simulink model "code_gen_man_bin_test"  (Simulink 7.5)
settings: Solver=FixedStepDiscrete  StartTime=0.0  StopTime=15  RelTol=1e-3
libraries: simulink x3
settings Model: Creator=Bryant  LastModifiedBy=Bryant

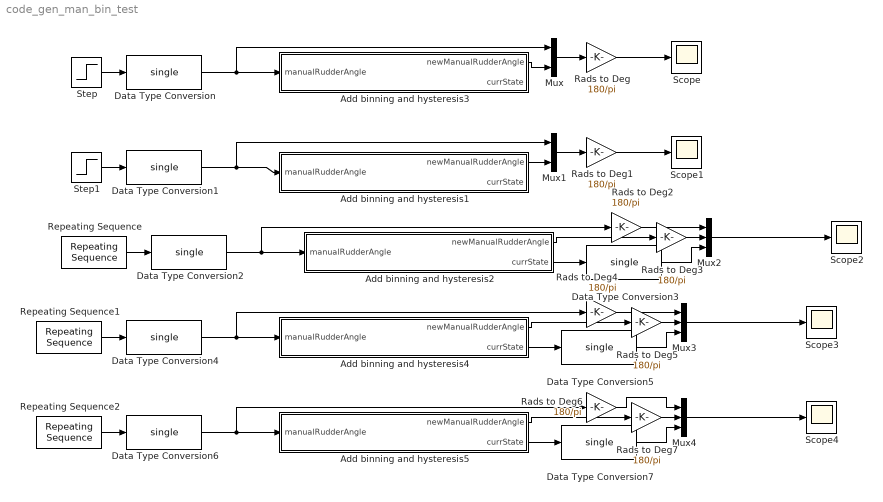
== system code_gen_man_bin_test ==
  Add binning and hysteresis1 : Stateflow chart  TreatAsAtomicUnit=on
  Add binning and hysteresis2 : Stateflow chart  TreatAsAtomicUnit=on
  Add binning and hysteresis3 : Stateflow chart  TreatAsAtomicUnit=on
  Add binning and hysteresis4 : Stateflow chart  TreatAsAtomicUnit=on
  Add binning and hysteresis5 : Stateflow chart  TreatAsAtomicUnit=on
  Data Type Conversion{,1..7} (8 alike) : DataTypeConversion  OutDataTypeMode=single  OutDataType=fixdt(1, 16)  OutScaling=2^0  OutDataTypeStr=single
  Mux : Mux  Inputs=2
  Mux1 : Mux  Inputs=2
  Mux2 : Mux  Inputs=3
  Mux3 : Mux  Inputs=3
  Mux4 : Mux  Inputs=3
  Rads to Deg{,1..7} (8 alike) : Gain  Gain=180/pi  ParameterDataType=fixdt(1, 16)  ParameterScaling=2^0  OutDataType=fixdt(1, 16)  OutScaling=2^0
  Repeating Sequence : simulink/Sources/Repeating Sequence  SystemSampleTime=-1  rep_seq_t=[0 1 1 2 2]  rep_seq_y=[0 0 35 35 0]*pi/180
  Repeating Sequence1 : simulink/Sources/Repeating Sequence  SystemSampleTime=-1  rep_seq_t=[0 1 1 2 2]  rep_seq_y=[0 0 -35 -35 0]*pi/180
  Repeating Sequence2 : simulink/Sources/Repeating Sequence  SystemSampleTime=-1  rep_seq_t=[0 1 1 2 2 3 3 4 4 5 5 6 6]  rep_seq_y=[0 0 -35 -35 0 0 35 35 0 0 -35 -35 0]*pi/180
  Scope{,1..4} (5 alike) : Scope
      Scope2 settings: SaveName=ScopeData2
      Scope3 settings: SaveName=ScopeData3
      Scope4 settings: SaveName=ScopeData4
  Step : Step  After=35*pi/180  SampleTime=.01
  Step1 : Step  After=-35*pi/180  SampleTime=.01
  wires:
  Step/1 -> Data Type Conversion/1
  Add binning and hysteresis3/1(newManualRudderAngle) -> Mux/2
  Mux/1 -> Rads to Deg/1
  Data Type Conversion/1 -> Mux/1, Add binning and hysteresis3/1(manualRudderAngle)
  Rads to Deg/1 -> Scope/1
  Step1/1 -> Data Type Conversion1/1
  Add binning and hysteresis1/1(newManualRudderAngle) -> Mux1/2
  Mux1/1 -> Rads to Deg1/1
  Data Type Conversion1/1 -> Mux1/1, Add binning and hysteresis1/1(manualRudderAngle)
  Rads to Deg1/1 -> Scope1/1
  Add binning and hysteresis2/1(newManualRudderAngle) -> Rads to Deg3/1
  Mux2/1 -> Scope2/1
  Data Type Conversion2/1 -> Add binning and hysteresis2/1(manualRudderAngle), Rads to Deg2/1
  Repeating Sequence/1 -> Data Type Conversion2/1
  Add binning and hysteresis2/2(currState) -> Data Type Conversion3/1
  Data Type Conversion3/1 -> Mux2/3
  Rads to Deg2/1 -> Mux2/1
  Rads to Deg3/1 -> Mux2/2
  Add binning and hysteresis4/1(newManualRudderAngle) -> Rads to Deg5/1
  Mux3/1 -> Scope3/1
  Data Type Conversion4/1 -> Add binning and hysteresis4/1(manualRudderAngle), Rads to Deg4/1
  Repeating Sequence1/1 -> Data Type Conversion4/1
  Add binning and hysteresis4/2(currState) -> Data Type Conversion5/1
  Data Type Conversion5/1 -> Mux3/3
  Rads to Deg4/1 -> Mux3/1
  Rads to Deg5/1 -> Mux3/2
  Add binning and hysteresis5/1(newManualRudderAngle) -> Rads to Deg7/1
  Mux4/1 -> Scope4/1
  Data Type Conversion6/1 -> Add binning and hysteresis5/1(manualRudderAngle), Rads to Deg6/1
  Repeating Sequence2/1 -> Data Type Conversion6/1
  Add binning and hysteresis5/2(currState) -> Data Type Conversion7/1
  Data Type Conversion7/1 -> Mux4/3
  Rads to Deg7/1 -> Mux4/2
  Rads to Deg6/1 -> Mux4/1

== matlab function Add binning and hysteresis1 ==
  data: manualRudderAngle input double; newManualRudderAngle output double; currState output double
function [newManualRudderAngle,currState] = fcn(manualRudderAngle)
%#eml
    % This function converts the continuous input of the rudder angle
    % command into a up/down/no change control. This allows for the commanded
    % rudder value to remain constant, which is useful for doing rudder
    % tests.
    
    % Once the input is above 25 or below -25 degrees (in radians) then a
    % counter starts for 25 timesteps (so .25s total) to see if the rudder
    % angle should change. Then it waits until the commanded angle resets
    % to around 0 (between +- 10 degrees) and then another transition can
    % occur.
    
    % This function relies on a 4-state FSM. It follows the general pattern
    % of 0-1-3 or 0-2-3 on success. 0 is the initial state, 1 and 2 are the
    % same, just moving in different directions, and 3 is the cleanup.

    % Keep a counter going of how long they have requested a bin transition
    persistent transitionCounter state nullTransitionCounter;
    if isempty(transitionCounter)
        transitionCounter = uint8(0);
        nullTransitionCounter = uint8(0);
        state = uint8(0);
    end

    % Store the mapped rudder angles for each bin
    binAngles = single([-45 -33 -22 -11 0 11 22 33 45]*pi/180);

    % Keep track of which bin we're in so that hysteresis can be done. This is
    % NOT a stateless algorithm. We initialize into the 0th bin (which is 1 in
    % this case because of Matlab's 1 indexing).
    persistent bin;
    if isempty(bin)
        bin = uint8(5);
    end

    switch state
        case 0
            if manualRudderAngle > 25*pi/180;
                transitionCounter = uint8(0);
                state = uint8(1);
            elseif manualRudderAngle < -25*pi/180;
                transitionCounter = uint8(0);
                state = uint8(2);
            end
        case 1
            % If the user is still indicating a transition, keep counting.
            % Otherwise record null transition commands.
            if manualRudderAngle > 25*pi/180;
                transitionCounter = transitionCounter + uint8(1);
            else
                nullTransitionCounter = nullTransitionCounter + uint8(1);
            end
            
            % Either transition if possible and requested or fail out after
            % having encountered too many timesteps without a request.
            if transitionCounter > 25
                if bin + uint8(1) <= length(binAngles)
                    bin = bin + uint8(1);
                end
                state = uint8(3);
            elseif nullTransitionCounter > 8
                state = uint8(3);
            end
        case 2
            if manualRudderAngle < -25*pi/180;
                transitionCounter = transitionCounter + uint8(1);
            else
                nullTransitionCounter = nullTransitionCounter + uint8(1);
            end
            if transitionCounter > 25
                if bin - uint8(1) > 0
                    bin = bin - uint8(1);
                end
                state = uint8(3);
            elseif nullTransitionCounter > 8
                state = uint8(3);
            end
        case 3
            if manualRudderAngle < 10*pi/180 && manualRudderAngle > -10*pi/180
                state = uint8(0);
                nullTransitionCounter = uint8(0);
            end
    end
    
    newManualRudderAngle = binAngles(bin);
    currState = state;
end

== matlab function Add binning and hysteresis2 ==
  data: manualRudderAngle input double; newManualRudderAngle output double; currState output double
function [newManualRudderAngle,currState] = fcn(manualRudderAngle)
%#eml
    % This function converts the continuous input of the rudder angle
    % command into a up/down/no change control. This allows for the commanded
    % rudder value to remain constant, which is useful for doing rudder
    % tests.
    
    % Once the input is above 25 or below -25 degrees (in radians) then a
    % counter starts for 25 timesteps (so .25s total) to see if the rudder
    % angle should change. Then it waits until the commanded angle resets
    % to around 0 (between +- 10 degrees) and then another transition can
    % occur.
    
    % This function relies on a 4-state FSM. It follows the general pattern
    % of 0-1-3 or 0-2-3 on success. 0 is the initial state, 1 and 2 are the
    % same, just moving in different directions, and 3 is the cleanup.

    % Keep a counter going of how long they have requested a bin transition
    persistent transitionCounter state nullTransitionCounter;
    if isempty(transitionCounter)
        transitionCounter = uint8(0);
        nullTransitionCounter = uint8(0);
        state = uint8(0);
    end

    % Store the mapped rudder angles for each bin
    binAngles = single([-45 -33 -22 -11 0 11 22 33 45]*pi/180);

    % Keep track of which bin we're in so that hysteresis can be done. This is
    % NOT a stateless algorithm. We initialize into the 0th bin (which is 1 in
    % this case because of Matlab's 1 indexing).
    persistent bin;
    if isempty(bin)
        bin = uint8(5);
    end

    switch state
        case 0
            if manualRudderAngle > 25*pi/180;
                transitionCounter = uint8(0);
                state = uint8(1);
            elseif manualRudderAngle < -25*pi/180;
                transitionCounter = uint8(0);
                state = uint8(2);
            end
        case 1
            % If the user is still indicating a transition, keep counting.
            % Otherwise record null transition commands.
            if manualRudderAngle > 25*pi/180;
                transitionCounter = transitionCounter + uint8(1);
            else
                nullTransitionCounter = nullTransitionCounter + uint8(1);
            end
            
            % Either transition if possible and requested or fail out after
            % having encountered too many timesteps without a request.
            if transitionCounter > 25
                if bin + uint8(1) <= length(binAngles)
                    bin = bin + uint8(1);
                end
                state = uint8(3);
            elseif nullTransitionCounter > 8
                state = uint8(3);
            end
        case 2
            if manualRudderAngle < -25*pi/180;
                transitionCounter = transitionCounter + uint8(1);
            else
                nullTransitionCounter = nullTransitionCounter + uint8(1);
            end
            if transitionCounter > 25
                if bin - uint8(1) > 0
                    bin = bin - uint8(1);
                end
                state = uint8(3);
            elseif nullTransitionCounter > 8
                state = uint8(3);
            end
        case 3
            if manualRudderAngle < 10*pi/180 && manualRudderAngle > -10*pi/180
                state = uint8(0);
                nullTransitionCounter = uint8(0);
            end
    end
    
    newManualRudderAngle = binAngles(bin);
    currState = state;
end

== matlab function Add binning and hysteresis3 ==
  data: manualRudderAngle input double; newManualRudderAngle output double; currState output double
function [newManualRudderAngle,currState] = fcn(manualRudderAngle)
%#eml
    % This function converts the continuous input of the rudder angle
    % command into a up/down/no change control. This allows for the commanded
    % rudder value to remain constant, which is useful for doing rudder
    % tests.
    
    % Once the input is above 25 or below -25 degrees (in radians) then a
    % counter starts for 25 timesteps (so .25s total) to see if the rudder
    % angle should change. Then it waits until the commanded angle resets
    % to around 0 (between +- 10 degrees) and then another transition can
    % occur.
    
    % This function relies on a 4-state FSM. It follows the general pattern
    % of 0-1-3 or 0-2-3 on success. 0 is the initial state, 1 and 2 are the
    % same, just moving in different directions, and 3 is the cleanup.

    % Keep a counter going of how long they have requested a bin transition
    persistent transitionCounter state nullTransitionCounter;
    if isempty(transitionCounter)
        transitionCounter = uint8(0);
        nullTransitionCounter = uint8(0);
        state = uint8(0);
    end

    % Store the mapped rudder angles for each bin
    binAngles = single([-45 -33 -22 -11 0 11 22 33 45]*pi/180);

    % Keep track of which bin we're in so that hysteresis can be done. This is
    % NOT a stateless algorithm. We initialize into the 0th bin (which is 1 in
    % this case because of Matlab's 1 indexing).
    persistent bin;
    if isempty(bin)
        bin = uint8(5);
    end

    switch state
        case 0
            if manualRudderAngle > 25*pi/180;
                transitionCounter = uint8(0);
                state = uint8(1);
            elseif manualRudderAngle < -25*pi/180;
                transitionCounter = uint8(0);
                state = uint8(2);
            end
        case 1
            % If the user is still indicating a transition, keep counting.
            % Otherwise record null transition commands.
            if manualRudderAngle > 25*pi/180;
                transitionCounter = transitionCounter + uint8(1);
            else
                nullTransitionCounter = nullTransitionCounter + uint8(1);
            end
            
            % Either transition if possible and requested or fail out after
            % having encountered too many timesteps without a request.
            if transitionCounter > 25
                if bin + uint8(1) <= length(binAngles)
                    bin = bin + uint8(1);
                end
                state = uint8(3);
            elseif nullTransitionCounter > 8
                state = uint8(3);
            end
        case 2
            if manualRudderAngle < -25*pi/180;
                transitionCounter = transitionCounter + uint8(1);
            else
                nullTransitionCounter = nullTransitionCounter + uint8(1);
            end
            if transitionCounter > 25
                if bin - uint8(1) > 0
                    bin = bin - uint8(1);
                end
                state = uint8(3);
            elseif nullTransitionCounter > 8
                state = uint8(3);
            end
        case 3
            if manualRudderAngle < 10*pi/180 && manualRudderAngle > -10*pi/180
                state = uint8(0);
                nullTransitionCounter = uint8(0);
            end
    end
    
    newManualRudderAngle = binAngles(bin);
    currState = state;
end

== matlab function Add binning and hysteresis4 ==
  data: manualRudderAngle input double; newManualRudderAngle output double; currState output double
function [newManualRudderAngle,currState] = fcn(manualRudderAngle)
%#eml
    % This function converts the continuous input of the rudder angle
    % command into a up/down/no change control. This allows for the commanded
    % rudder value to remain constant, which is useful for doing rudder
    % tests.
    
    % Once the input is above 25 or below -25 degrees (in radians) then a
    % counter starts for 25 timesteps (so .25s total) to see if the rudder
    % angle should change. Then it waits until the commanded angle resets
    % to around 0 (between +- 10 degrees) and then another transition can
    % occur.
    
    % This function relies on a 4-state FSM. It follows the general pattern
    % of 0-1-3 or 0-2-3 on success. 0 is the initial state, 1 and 2 are the
    % same, just moving in different directions, and 3 is the cleanup.

    % Keep a counter going of how long they have requested a bin transition
    persistent transitionCounter state nullTransitionCounter;
    if isempty(transitionCounter)
        transitionCounter = uint8(0);
        nullTransitionCounter = uint8(0);
        state = uint8(0);
    end

    % Store the mapped rudder angles for each bin
    binAngles = single([-45 -33 -22 -11 0 11 22 33 45]*pi/180);

    % Keep track of which bin we're in so that hysteresis can be done. This is
    % NOT a stateless algorithm. We initialize into the 0th bin (which is 1 in
    % this case because of Matlab's 1 indexing).
    persistent bin;
    if isempty(bin)
        bin = uint8(5);
    end

    switch state
        case 0
            if manualRudderAngle > 25*pi/180;
                transitionCounter = uint8(0);
                state = uint8(1);
            elseif manualRudderAngle < -25*pi/180;
                transitionCounter = uint8(0);
                state = uint8(2);
            end
        case 1
            % If the user is still indicating a transition, keep counting.
            % Otherwise record null transition commands.
            if manualRudderAngle > 25*pi/180;
                transitionCounter = transitionCounter + uint8(1);
            else
                nullTransitionCounter = nullTransitionCounter + uint8(1);
            end
            
            % Either transition if possible and requested or fail out after
            % having encountered too many timesteps without a request.
            if transitionCounter > 25
                if bin + uint8(1) <= length(binAngles)
                    bin = bin + uint8(1);
                end
                state = uint8(3);
            elseif nullTransitionCounter > 8
                state = uint8(3);
            end
        case 2
            if manualRudderAngle < -25*pi/180;
                transitionCounter = transitionCounter + uint8(1);
            else
                nullTransitionCounter = nullTransitionCounter + uint8(1);
            end
            if transitionCounter > 25
                if bin - uint8(1) > 0
                    bin = bin - uint8(1);
                end
                state = uint8(3);
            elseif nullTransitionCounter > 8
                state = uint8(3);
            end
        case 3
            if manualRudderAngle < 10*pi/180 && manualRudderAngle > -10*pi/180
                state = uint8(0);
                nullTransitionCounter = uint8(0);
            end
    end
    
    newManualRudderAngle = binAngles(bin);
    currState = state;
end

== matlab function Add binning and hysteresis5 ==
  data: manualRudderAngle input double; newManualRudderAngle output double; currState output double
function [newManualRudderAngle,currState] = fcn(manualRudderAngle)
%#eml
    % This function converts the continuous input of the rudder angle
    % command into a up/down/no change control. This allows for the commanded
    % rudder value to remain constant, which is useful for doing rudder
    % tests.
    
    % Once the input is above 25 or below -25 degrees (in radians) then a
    % counter starts for 25 timesteps (so .25s total) to see if the rudder
    % angle should change. Then it waits until the commanded angle resets
    % to around 0 (between +- 10 degrees) and then another transition can
    % occur.
    
    % This function relies on a 4-state FSM. It follows the general pattern
    % of 0-1-3 or 0-2-3 on success. 0 is the initial state, 1 and 2 are the
    % same, just moving in different directions, and 3 is the cleanup.

    % Keep a counter going of how long they have requested a bin transition
    persistent transitionCounter state nullTransitionCounter;
    if isempty(transitionCounter)
        transitionCounter = uint8(0);
        nullTransitionCounter = uint8(0);
        state = uint8(0);
    end

    % Store the mapped rudder angles for each bin
    binAngles = single([-45 -33 -22 -11 0 11 22 33 45]*pi/180);

    % Keep track of which bin we're in so that hysteresis can be done. This is
    % NOT a stateless algorithm. We initialize into the 0th bin (which is 1 in
    % this case because of Matlab's 1 indexing).
    persistent bin;
    if isempty(bin)
        bin = uint8(5);
    end

    switch state
        case 0
            if manualRudderAngle > 25*pi/180;
                transitionCounter = uint8(0);
                state = uint8(1);
            elseif manualRudderAngle < -25*pi/180;
                transitionCounter = uint8(0);
                state = uint8(2);
            end
        case 1
            % If the user is still indicating a transition, keep counting.
            % Otherwise record null transition commands.
            if manualRudderAngle > 25*pi/180;
                transitionCounter = transitionCounter + uint8(1);
            else
                nullTransitionCounter = nullTransitionCounter + uint8(1);
            end
            
            % Either transition if possible and requested or fail out after
            % having encountered too many timesteps without a request.
            if transitionCounter > 25
                if bin + uint8(1) <= length(binAngles)
                    bin = bin + uint8(1);
                end
                state = uint8(3);
            elseif nullTransitionCounter > 8
                state = uint8(3);
            end
        case 2
            if manualRudderAngle < -25*pi/180;
                transitionCounter = transitionCounter + uint8(1);
            else
                nullTransitionCounter = nullTransitionCounter + uint8(1);
            end
            if transitionCounter > 25
                if bin - uint8(1) > 0
                    bin = bin - uint8(1);
                end
                state = uint8(3);
            elseif nullTransitionCounter > 8
                state = uint8(3);
            end
        case 3
            if manualRudderAngle < 10*pi/180 && manualRudderAngle > -10*pi/180
                state = uint8(0);
                nullTransitionCounter = uint8(0);
            end
    end
    
    newManualRudderAngle = binAngles(bin);
    currState = state;
end
